simulink model "Copy_of_Facies"  (R2023a)
settings: Solver=VariableStepAuto  StartTime=0.0  StopTime=6  RelTol=1e-3
(part 2 of 2)

== matlab function Copy_of_Facies/media ==
  data: u input; y output
function y = media(u)

y = mean(u);

== matlab function Copy_of_Facies/media2 ==
  data: u input; y output
function y = media(u)

y = mean(u);

== matlab function Copy_of_Facies/media1 ==
  data: u input; y output
function y = media(u)

y = mean(u);
